simulink model "drone_nonlinear_full_control"  (R2018a)
settings: Solver=VariableStepAuto  StartTime=0.0  StopTime=20  RelTol=1e-3
undefined symbols (not defined in the file): est_c_A, est_c_B, est_c_C, est_c_D, est_c_K, g, Ix, Iy, Iz, m, obs_c_L, simulation_sampling_ts
settings Model: Creator=ros  LastModifiedBy=ros

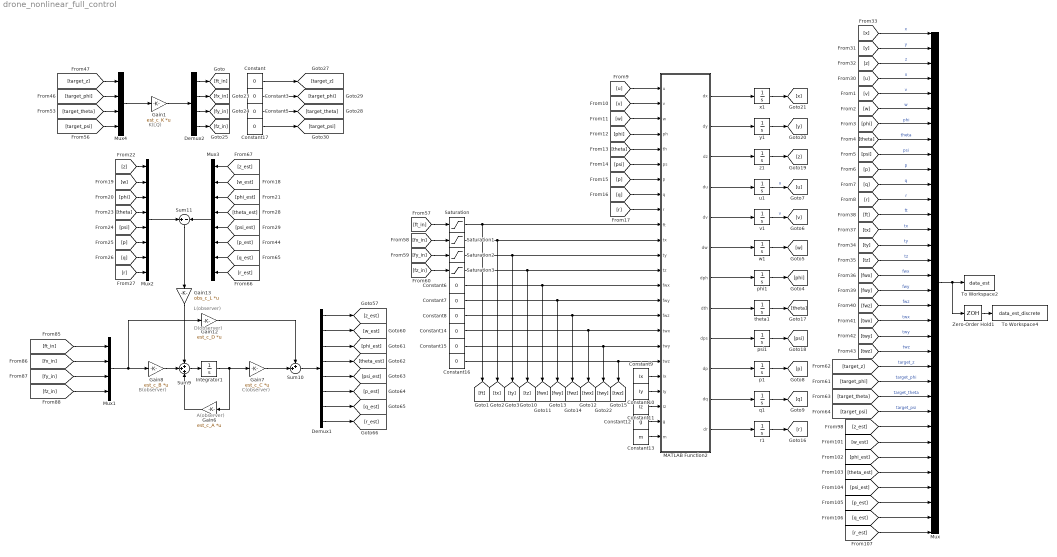
== system drone_nonlinear_full_control ==
  note: B(observer)
  note: C(observer)
  note: A(observer)
  note: D(observer)
  note: L(observer)
  note: K(LQ)
  Constant{,3,5..8,14..17} (10 alike) : Constant  Value=0
  Constant10 : Constant  Value=Iy
  Constant11 : Constant  Value=Iz
  Constant12 : Constant  Value=g
  Constant13 : Constant  Value=m
  Constant9 : Constant  Value=Ix
  Demux1 : Demux  Outputs=8
  Demux2 : Demux
  Gain1 : Gain  Gain=est_c_K  Multiplication=Matrix(K*u)
  Gain12 : Gain  Gain=est_c_D  Multiplication=Matrix(K*u)
  Gain13 : Gain  Gain=obs_c_L  Multiplication=Matrix(K*u)
  Gain6 : Gain  Gain=est_c_A  Multiplication=Matrix(K*u)
  Gain7 : Gain  Gain=est_c_C  Multiplication=Matrix(K*u)
  Gain8 : Gain  Gain=est_c_B  Multiplication=Matrix(K*u)
  Integrator1 : Integrator
  MATLAB Function2 : MATLAB Function  TreatAsAtomicUnit=on
  Mux : Mux  Inputs=34
  Mux1 : Mux
  Mux2 : Mux  Inputs=8
  Mux3 : Mux  Inputs=8
  Mux4 : Mux
  Saturation{,1..3} (4 alike) : Saturate  UpperLimit=30  LowerLimit=-100
  Sum10 : Sum  Inputs=++|
  Sum11 : Sum  Inputs=+-
  Sum9 : Sum  Inputs=+++
  To Workspace2 : ToWorkspace  VariableName=data_est  SaveFormat=Timeseries  SampleTime=-1
  To Workspace4 : ToWorkspace  VariableName=data_est_discrete  SaveFormat=Timeseries  SampleTime=-1
  Zero-Order Hold1 : ZeroOrderHold  SampleTime=simulation_sampling_ts
  p1 : Integrator
  phi1 : Integrator
  psi1 : Integrator
  q1 : Integrator
  r1 : Integrator
  theta1 : Integrator
  u1 : Integrator
  v1 : Integrator
  w1 : Integrator
  x1 : Integrator
  y1 : Integrator
  z1 : Integrator
  wires:
  [v] -> MATLAB Function2/2(v)
  MATLAB Function2/9(dps) -> psi1/1
  MATLAB Function2/10(dp) -> p1/1
  MATLAB Function2/5(dv) -> v1/1
  [r] -> MATLAB Function2/9(r)
  [psi] -> MATLAB Function2/6(ps)
  [p] -> MATLAB Function2/7(p)
  p1/1 -> [p]
  MATLAB Function2/12(dr) -> r1/1
  theta1/1 -> [theta]
  [w] -> MATLAB Function2/3(w)
  [phi] -> MATLAB Function2/4(ph)
  [q] -> MATLAB Function2/8(q)
  r1/1 -> [r]
  q1/1 -> [q]
  MATLAB Function2/11(dq) -> q1/1
  MATLAB Function2/6(dw) -> w1/1
  MATLAB Function2/4(du) -> u1/1
  psi1/1 -> [psi]
  [u] -> MATLAB Function2/1(u)
  MATLAB Function2/8(dth) -> theta1/1
  [theta] -> MATLAB Function2/5(th)
  u1/1 -> [u]  "u"
  w1/1 -> [w]
  MATLAB Function2/7(dph) -> phi1/1
  v1/1 -> [v]  "v"
  Constant9/1 -> MATLAB Function2/20(Ix)
  Constant13/1 -> MATLAB Function2/24(m)
  Constant11/1 -> MATLAB Function2/22(Iz)
  Constant10/1 -> MATLAB Function2/21(Iy)
  Constant12/1 -> MATLAB Function2/23(g)
  MATLAB Function2/1(dx) -> x1/1
  MATLAB Function2/2(dy) -> y1/1
  MATLAB Function2/3(dz) -> z1/1
  Constant6/1 -> [fwx], MATLAB Function2/14(fwx)
  Constant7/1 -> [fwy], MATLAB Function2/15(fwy)
  Constant14/1 -> [twx], MATLAB Function2/17(twx)
  Constant8/1 -> [fwz], MATLAB Function2/16(fwz)
  Constant15/1 -> [twy], MATLAB Function2/18(twy)
  Constant16/1 -> [twz], MATLAB Function2/19(twz)
  z1/1 -> [z]
  y1/1 -> [y]
  x1/1 -> [x]
  [x] -> Mux/1  "x"
  [v] -> Mux/5  "v"
  [z] -> Mux/3  "z"
  [w] -> Mux/6  "w"
  [p] -> Mux/10  "p"
  [phi] -> Mux/7  "phi"
  [theta] -> Mux/8  "theta"
  [r] -> Mux/12  "r"
  [y] -> Mux/2  "y"
  [psi] -> Mux/9  "psi"
  [u] -> Mux/4  "u"
  [q] -> Mux/11  "q"
  Mux/1 -> Zero-Order Hold1/1, To Workspace2/1
  [ft] -> Mux/13  "ft"
  [tx] -> Mux/14  "tx"
  [ty] -> Mux/15  "ty"
  [tz] -> Mux/16  "tz"
  [fwx] -> Mux/17  "fwx"
  [fwy] -> Mux/18  "fwy"
  [fwz] -> Mux/19  "fwz"
  [twx] -> Mux/20  "twx"
  [twy] -> Mux/21  "twy"
  [twz] -> Mux/22  "twz"
  phi1/1 -> [phi]
  Zero-Order Hold1/1 -> To Workspace4/1
  Saturation/1 -> [ft], MATLAB Function2/10(ft)
  Saturation1/1 -> [tx], MATLAB Function2/11(tx)
  Saturation2/1 -> [ty], MATLAB Function2/12(ty)
  Saturation3/1 -> [tz], MATLAB Function2/13(tz)
  [target_z] -> Mux/23  "target_z"
  [target_phi] -> Mux/24  "target_phi"
  [target_theta] -> Mux/25  "target_theta"
  [target_psi] -> Mux/26  "target_psi"
  [ft_in] -> Saturation/1
  [fx_in] -> Saturation1/1
  [fy_in] -> Saturation2/1
  [fz_in] -> Saturation3/1
  Constant17/1 -> [target_psi]
  Constant5/1 -> [target_theta]
  Constant/1 -> [target_z]
  Constant3/1 -> [target_phi]
  Mux1/1 -> Gain12/1, Gain8/1
  Sum9/1 -> Integrator1/1
  Integrator1/1 -> Gain7/1, Gain6/1
  Gain8/1 -> Sum9/2
  Gain6/1 -> Sum9/3
  Gain7/1 -> Sum10/2
  [fz_in] -> Mux1/4
  [fx_in] -> Mux1/2
  [ft_in] -> Mux1/1
  [fy_in] -> Mux1/3
  Gain12/1 -> Sum10/1
  Sum10/1 -> Demux1/1
  Demux1/1 -> [z_est]
  Demux1/2 -> [w_est]
  Demux1/3 -> [phi_est]
  Demux1/4 -> [theta_est]
  Demux1/5 -> [psi_est]
  Demux1/6 -> [p_est]
  Demux1/7 -> [q_est]
  Demux1/8 -> [r_est]
  [z] -> Mux2/1
  [w] -> Mux2/2
  [phi] -> Mux2/3
  [theta] -> Mux2/4
  [psi] -> Mux2/5
  [p] -> Mux2/6
  [q] -> Mux2/7
  [r] -> Mux2/8
  Gain13/1 -> Sum9/1
  [z_est] -> Mux3/1
  [w_est] -> Mux3/2
  [phi_est] -> Mux3/3
  [theta_est] -> Mux3/4
  [psi_est] -> Mux3/5
  [p_est] -> Mux3/6
  [q_est] -> Mux3/7
  [r_est] -> Mux3/8
  Mux3/1 -> Sum11/2
  Mux2/1 -> Sum11/1
  Sum11/1 -> Gain13/1
  [target_z] -> Mux4/1
  [target_phi] -> Mux4/2
  [target_theta] -> Mux4/3
  [target_psi] -> Mux4/4
  Mux4/1 -> Gain1/1
  [z_est] -> Mux/27
  [w_est] -> Mux/28
  [phi_est] -> Mux/29
  [theta_est] -> Mux/30
  [psi_est] -> Mux/31
  [p_est] -> Mux/32
  [q_est] -> Mux/33
  [r_est] -> Mux/34
  Gain1/1 -> Demux2/1
  Demux2/1 -> [ft_in]
  Demux2/2 -> [fx_in]
  Demux2/3 -> [fy_in]
  Demux2/4 -> [fz_in]

== matlab function drone_nonlinear_full_control/MATLAB Function2 ==
  data: u input; v input; dx output; w input; ph input; th input; ps input; p input; q input; r input; ft input; tx input; ty input; tz input; fwx input; fwy input; fwz input; twx input; twy input; twz input; dy output; dz output; du output; dv output; dw output; dph output; dth output; dps output; dp output; dq output; dr output; Ix input; Iy input; Iz input; g input; m input
function [dx, dy, dz, du, dv, dw, dph, dth, dps, dp, dq, dr] = fcn(u, v, w, ph, th, ps, p, q, r, ft, tx, ty, tz, fwx, fwy, fwz, twx, twy, twz, Ix, Iy, Iz, g, m)

dx = w*(sin(ph)*sin(ps) + cos(ph)*cos(ps)*sin(th)) - v*(cos(ph)*sin(ps) - cos(ps)*sin(ph)*sin(th)) + u*(cos(ps)*cos(th));
dy = v*(cos(ph)*cos(ps) + sin(ph)*sin(ps)*sin(th)) - w*(cos(ps)*sin(ph) - cos(ph)*sin(ps)*sin(th)) + u*(cos(th)*sin(ps));
dz = w*(cos(ph)*cos(th)) - u*(sin(th)) + v*(cos(th)*sin(ph));
du = r*v - q*w + g*(sin(th)) + fwx / m;
dv = p*w - r*u - g*(sin(ph)*cos(th)) + fwy / m;
dw = q*u - p*v - g*(cos(th)*cos(ph)) + (fwz + ft) / m;
dph = p + r*(cos(ph)*tan(th)) + q*(sin(ph)*tan(th));
dth = q*(cos(th)) - r*(sin(ph));
dps = r*(cos(ph)/cos(th)) + q*(sin(ph)/cos(th));
dp = r*q*(Iy - Iz)/Ix + (tx + twx)/Ix;
dq = p*r*(Iz - Ix)/Iy + (ty + twy)/Iy;
dr = p*q*(Ix - Iy)/Iz + (tz + twz)/Iz;
